simulink model "mnist_softmax"  (R2017a)
settings: Solver=FixedStepDiscrete  StartTime=0.0  StopTime=1000  FixedStep=1  RelTol=1e-3
undefined symbols (not defined in the file or in its folder): DiscIntNeverNeededParam
libraries: ad_blocks x7
settings Model: SimulationMode=accelerator  Creator=percro2  LastModifiedBy=eruffaldi

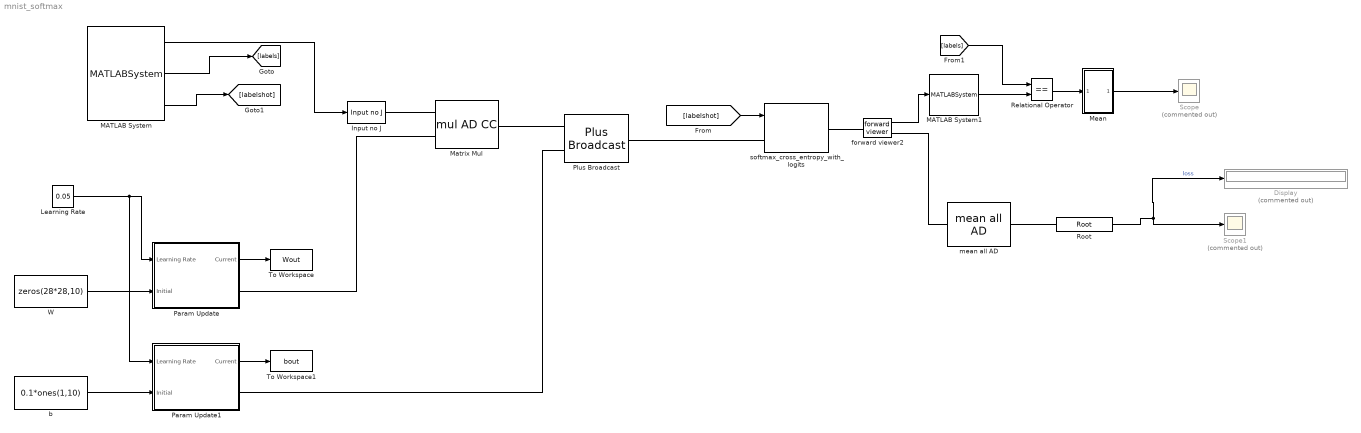
== system mnist_softmax ==
  Display : Display  Commented=on
  Input no J : ad_blocks/Input no J  SystemSampleTime=-1
  Learning Rate : Constant  Value=0.05
  MATLAB System : MATLABSystem  System=MnistSystemInt  trainset=1  items=100  SimulateUsing=Interpreted execution
      mask Type: MnistSystemInt
      mask Display:
      | disp('MnistSystemInt');
      | port_label('output',1,'x');
      | port_label('output',2,'labels');
      | port_label('output',3,'labelshot');
  MATLAB System1 : MATLABSystem  System=ArgmaxSystem  dim=2  SimulateUsing=Code generation
      mask Type: ArgmaxSystem
      mask Display:
      | disp('ArgmaxSystem');
      | port_label('input',1,'x');
      | port_label('output',1,'y');
  Matrix Mul : ad_blocks/mul AD CC
  Mean : Subsystem
  Param Update : Subsystem
  Param Update1 : Subsystem
  Plus Broadcast : ad_blocks/Plus Broadcast
  Relational Operator : RelationalOperator  Operator===  OutDataTypeStr=boolean  RndMeth=Simplest
  Root : ad_blocks/Root  Description=Top level AD block: gets the incoming value, pushes the scalar 1 gradient  SystemSampleTime=-1
  Scope : Scope  Commented=on
  Scope1 : Scope  Commented=on
  To Workspace : ToWorkspace  VariableName=Wout  SaveFormat=Timeseries  SampleTime=-1
  To Workspace1 : ToWorkspace  VariableName=bout  SaveFormat=Timeseries  SampleTime=-1
  W : Constant  Value=zeros(28*28,10)
  b : Constant  Value=0.1*ones(1,10)
  forward viewer2 : ad_blocks/forward viewer  SystemSampleTime=-1
  mean all AD : ad_blocks/mean all AD
  softmax_cross_entropy_with_logits : ad_blocks/softmax_cross_entropy_with_logits
  wires:
  MATLAB System/1 -> Input no J/1
  Root/1 -> Display/1, Scope1/1  "loss"
  forward viewer2/1 -> MATLAB System1/1
  Learning Rate/1 -> Param Update1/1(Learning Rate), Param Update/1(Learning Rate)
  W/1 -> Param Update/2(Initial)
  Param Update/1(Current) -> To Workspace/1
  Param Update1/1(Current) -> To Workspace1/1
  MATLAB System1/1 -> Relational Operator/2
  MATLAB System/2 -> [labels]
  [labelshot] -> softmax_cross_entropy_with_logits/1
  [labels] -> Relational Operator/1
  MATLAB System/3 -> [labelshot]
  b/1 -> Param Update1/2(Initial)
  Mean/1(Out1) -> Scope/1
  Relational Operator/1 -> Mean/1(In1)
  connections:
  Input no J/RConn1 -- Matrix Mul/LConn1
  Param Update/RConn1 -- Matrix Mul/LConn2
  Param Update1/RConn1 -- Plus Broadcast/LConn2
  Plus Broadcast/RConn1 -- softmax_cross_entropy_with_logits/LConn1
  softmax_cross_entropy_with_logits/RConn1 -- forward viewer2/LConn1
  mean all AD/RConn1 -- Root/LConn1
  forward viewer2/RConn1 -- mean all AD/LConn1
  Matrix Mul/RConn1 -- Plus Broadcast/LConn1

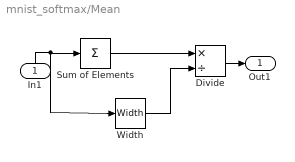
== system mnist_softmax/Mean ==
  In1 : Inport
  Divide : Product  Inputs=*/
  Sum of Elements : Sum  Inputs=+
  Width : Width
  Out1 : Outport
  wires:
  Divide/1 -> Out1/1
  In1/1 -> Width/1, Sum of Elements/1
  Sum of Elements/1 -> Divide/1
  Width/1 -> Divide/2

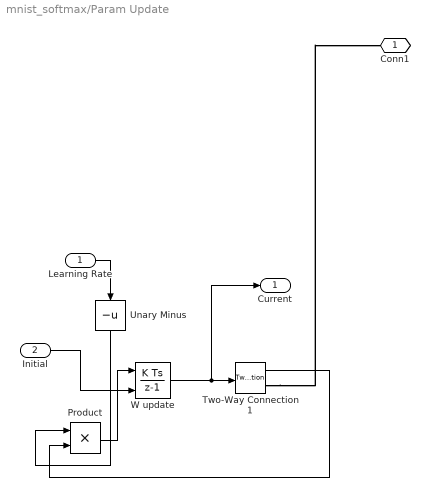
== system mnist_softmax/Param Update ==
  Learning Rate : Inport
  Initial : Inport  Port=2
  Product : Product
  Two-Way Connection1 : TwoWayConnection
  Unary Minus : UnaryMinus
  W update : DiscreteIntegrator  InitialConditionSource=external  InitialConditionSetting=State (most efficient)  SampleTime=-1  ICPrevOutput=DiscIntNeverNeededParam  ICPrevScaledInput=DiscIntNeverNeededParam
  Conn1 : PMIOPort  Port=1  Side=Right
  Current : Outport
  wires:
  Learning Rate/1 -> Unary Minus/1
  Product/1 -> W update/1
  Initial/1 -> W update/2
  Two-Way Connection1/1 -> Product/2
  W update/1 -> Current/1, Two-Way Connection1/1
  Unary Minus/1 -> Product/1
  connections:
  Two-Way Connection1/RConn1 -- Conn1/RConn1

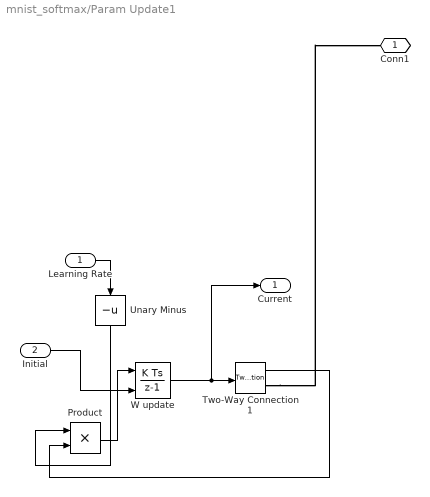
== system mnist_softmax/Param Update1 ==
  Learning Rate : Inport
  Initial : Inport  Port=2
  Product : Product
  Two-Way Connection1 : TwoWayConnection
  Unary Minus : UnaryMinus
  W update : DiscreteIntegrator  InitialConditionSource=external  InitialConditionSetting=State (most efficient)  SampleTime=-1  ICPrevOutput=DiscIntNeverNeededParam  ICPrevScaledInput=DiscIntNeverNeededParam
  Conn1 : PMIOPort  Port=1  Side=Right
  Current : Outport
  wires:
  Learning Rate/1 -> Unary Minus/1
  Product/1 -> W update/1
  Initial/1 -> W update/2
  Two-Way Connection1/1 -> Product/2
  W update/1 -> Current/1, Two-Way Connection1/1
  Unary Minus/1 -> Product/1
  connections:
  Two-Way Connection1/RConn1 -- Conn1/RConn1
